simulink model "task_4_sim"  (R2022b)
settings: Solver=VariableStepAuto  StartTime=0.0  StopTime=50.0  FixedStep=0.5  RelTol=1e-3
model workspace (MAT data in the model file):
  C0 = [1  0  0  0  0  0; 0  1  0  0  0  0; 0  0  1  0  0  0; 0  0  0  1  0  0; 0  0  0  0  1  0; 0  0  0  0  0  1]
  D0 = [0  0; 0  0; 0  0; 0  0; 0  0; 0  0]
values from neighbouring files (symbols this model uses):
  A = [-1 1 0 ... (first row only)    [test.m]
  B = [1 1 ... (first row only)    [test.m]
  C4 = [1 0 0 0 0 0 ... (first row only)    [task4.m]
  F4_1 = inv(BStar)    [task4.m]
  K4_2 = inv(BStar)*CStarStar    [task4.m]
  x0 = [0, 0, 0, 0, 0, 0]    [test.m]
settings Model: Creator=小灰  LastModifiedBy=小灰

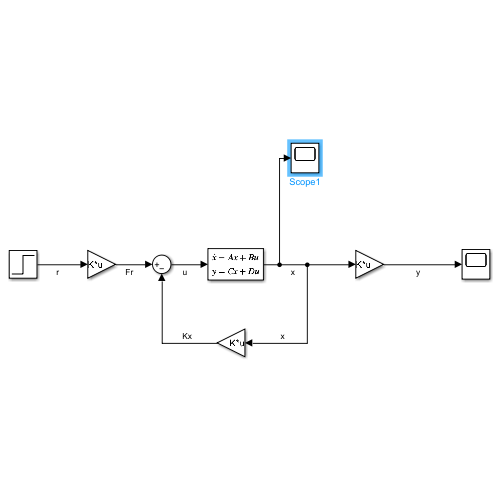
[thumbnail: Simulink's stored preview of the top-level diagram]
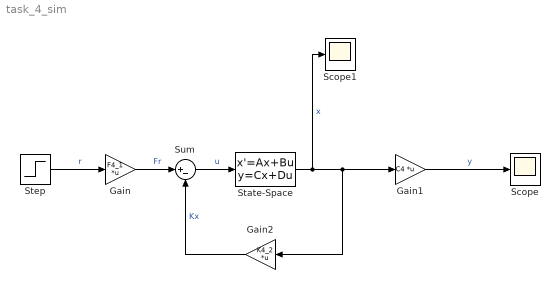
== system task_4_sim ==
  Gain : Gain  Gain=F4_1  Multiplication=Matrix(K*u)
  Gain1 : Gain  Gain=C4  Multiplication=Matrix(K*u)
  Gain2 : Gain  Gain=K4_2  Multiplication=Matrix(K*u)
  Scope : Scope
  Scope1 : Scope
  State-Space : StateSpace  A=A  B=B  C=C0  D=D0  InitialCondition=x0
  Step : Step  Time=2  Before=[0 0]  After=[0 0]  SampleTime=0
  Sum : Sum  Inputs=|+-
  wires:
  State-Space/1 -> Scope1/1, Gain2/1, Gain1/1  "x"
  Step/1 -> Gain/1  "r"
  Sum/1 -> State-Space/1  "u"
  Gain/1 -> Sum/1  "Fr"
  Gain2/1 -> Sum/2  "Kx"
  Gain1/1 -> Scope/1  "y"
